simulink model "PID_simulink"  (R2025a)
settings: Solver=VariableStepAuto  StartTime=0.0  StopTime=10.0  RelTol=1e-3
undefined symbols (not defined in the file or in its folder): Kd1, Kd2, Ki1, Ki2, Kp1, Kp2
settings Model: Creator=j chandini gayathri  LastModifiedBy=j chandini gayathri

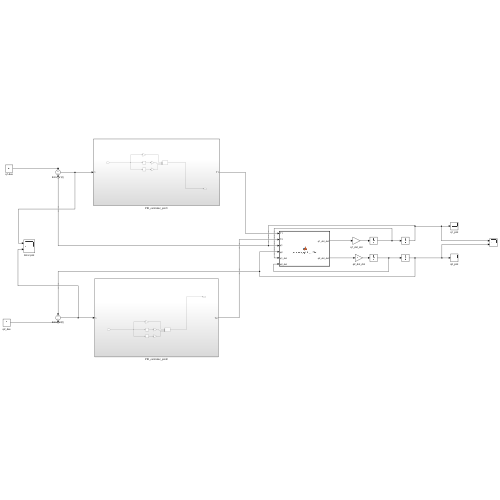
[thumbnail: Simulink's stored preview of the top-level diagram]
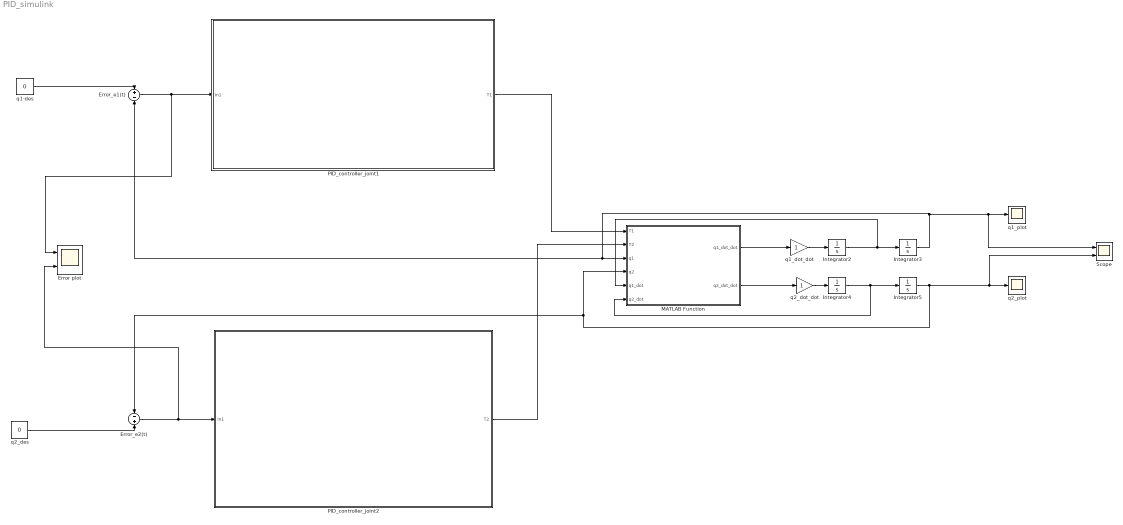
== system PID_simulink ==
  Error plot : Scope  NumInputPorts=2
      settings: Title=Ki_1= 5,Ki_2=5,Kp_1=200,Kp_2=200,Kd_1=400,Kd_2=400  ActiveDisplayYMinimum=-5.3633481280846287E+43  ActiveDisplayYMaximum=5.6403532247882645E+43  DataLoggingVariableName=ScopeData2
  Error_e1(t) : Sum  Inputs=+-
  Error_e2(t) : Sum  Inputs=-+
  Integrator{2..5} (4 alike) : Integrator
  MATLAB Function : MATLAB Function  TreatAsAtomicUnit=on
  PID_controller_joint1 : Subsystem
  PID_controller_joint2 : Subsystem
  Scope : Scope  NumInputPorts=2
      settings: ActiveDisplayYMinimum=-0.092497055065485209  ActiveDisplayYMaximum=0.011310468207808053  DataLoggingVariableName=ScopeData3
  q1-des : Constant  Value=0
  q1_dot_dot : Gain
  q1_plot : Scope
      settings: ActiveDisplayYMinimum=-0.092497055065485209  ActiveDisplayYMaximum=0.011310468207808053
  q2_des : Constant  Value=0
  q2_dot_dot : Gain
  q2_plot : Scope
      settings: ActiveDisplayYMinimum=-0.0028522802877235659  ActiveDisplayYMaximum=0.00045683308329411837
  wires:
  q1-des/1 -> Error_e1(t)/1
  Integrator2/1 -> MATLAB Function/5(q1_dot), Integrator3/1
  Integrator4/1 -> MATLAB Function/6(q2_dot), Integrator5/1
  Integrator3/1 -> Error_e1(t)/2, MATLAB Function/3(q1), Scope/1, q1_plot/1
  Integrator5/1 -> MATLAB Function/4(q2), Error_e2(t)/1, Scope/2, q2_plot/1
  q2_des/1 -> Error_e2(t)/2
  Error_e1(t)/1 -> Error plot/1, PID_controller_joint1/1(In1)
  Error_e2(t)/1 -> Error plot/2, PID_controller_joint2/1(In1)
  PID_controller_joint1/1(T1) -> MATLAB Function/1(T1)
  MATLAB Function/1(q1_dot_dot) -> q1_dot_dot/1
  MATLAB Function/2(q2_dot_dot) -> q2_dot_dot/1
  q1_dot_dot/1 -> Integrator2/1
  q2_dot_dot/1 -> Integrator4/1
  PID_controller_joint2/1(T2) -> MATLAB Function/2(T2)

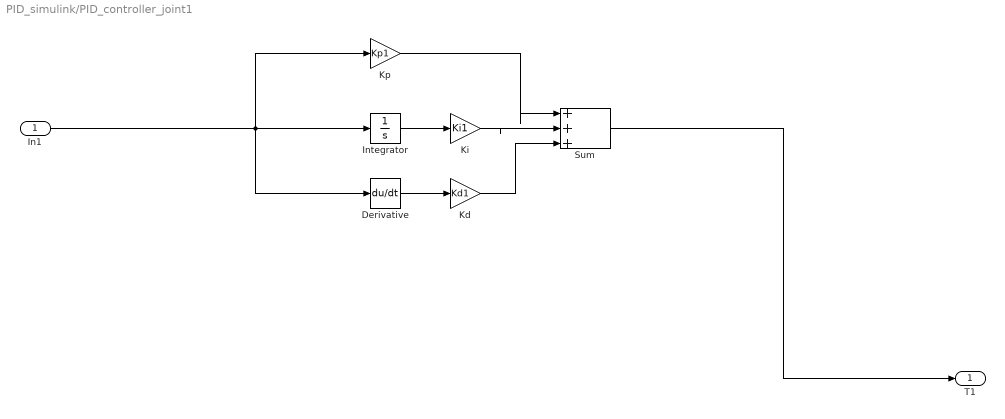
== system PID_simulink/PID_controller_joint1 ==
  In1 : Inport
  Derivative : Derivative
  Integrator : Integrator
  Kd : Gain  Gain=Kd1
  Ki : Gain  Gain=Ki1
  Kp : Gain  Gain=Kp1
  Sum : Sum  Inputs=|+++
  T1 : Outport
  wires:
  Kd/1 -> Sum/3
  Kp/1 -> Sum/1
  In1/1 -> Derivative/1, Kp/1, Integrator/1
  Derivative/1 -> Kd/1
  Sum/1 -> T1/1
  Integrator/1 -> Ki/1
  Ki/1 -> Sum/2

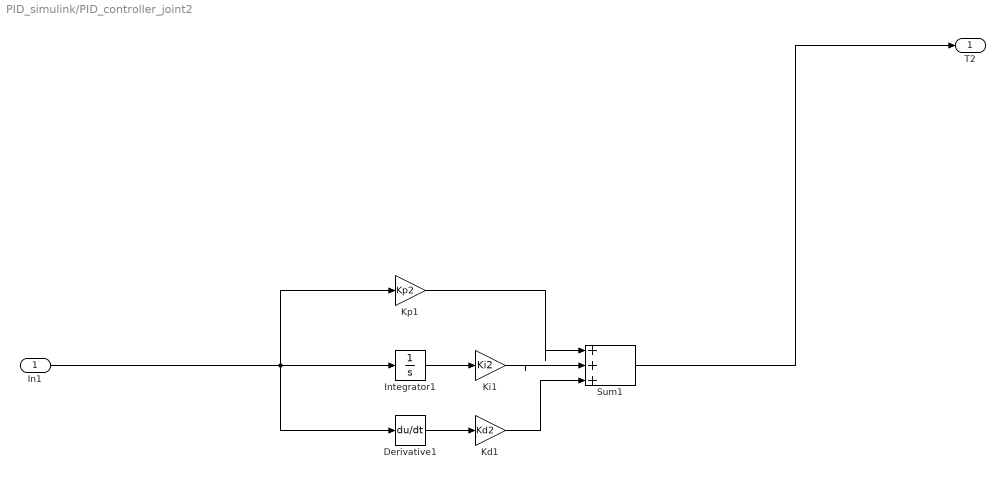
== system PID_simulink/PID_controller_joint2 ==
  In1 : Inport
  Derivative1 : Derivative
  Integrator1 : Integrator
  Kd1 : Gain  Gain=Kd2
  Ki1 : Gain  Gain=Ki2
  Kp1 : Gain  Gain=Kp2
  Sum1 : Sum  Inputs=|+++
  T2 : Outport
  wires:
  In1/1 -> Derivative1/1, Kp1/1, Integrator1/1
  Sum1/1 -> T2/1
  Kd1/1 -> Sum1/3
  Derivative1/1 -> Kd1/1
  Kp1/1 -> Sum1/1
  Ki1/1 -> Sum1/2
  Integrator1/1 -> Ki1/1

== matlab function PID_simulink/MATLAB Function ==
  data: T1 input; q1_dot_dot output; T2 input; q1 input; q2 input; q1_dot input; q2_dot input; q2_dot_dot output
function [q1_dot_dot, q2_dot_dot] = compute_q1dd_q2dd(T1, T2, q1, q2, q1_dot, q2_dot)
    m1 = 5; 
    m2 = 3;  
    l1 = 0.25; 
    l2 = 0.15; 
    g = 9.81; 
    M11 = (m1 + m2)*l1^2 + m2*l2*(l2 + 2*l1*cos(q2));
    M12=m2*l2*(l2 + l1*cos(q2));
    M21=m2*l2*(l2 + l1*cos(q2));
    M22=m2*l2^2;
    M=[M11 M12; M21 M22];
    C11 = -m2*l1*l2*sin(q2)*q2_dot;
    C12 = -m2*l1*l2*sin(q2)*(q1_dot + q2_dot);
    C21 = 0;
    C22 = m2*l1*l2*sin(q2)*q1_dot;
    C = [C11 C12; C21 C22];
    G1 = m1*l1*g*cos(q1) + m2*g*(l2*cos(q1 + q2) + l1*cos(q1));
    G2 = m2*g*l2*cos(q1 + q2);
    G = [G1; G2];
    tau = [T1; T2];
    q_dot = [q1_dot; q2_dot];
    q_dot_dot = (tau - (C*q_dot + G))./M;
    q1_dot_dot = q_dot_dot(1);
    q2_dot_dot = q_dot_dot(2);
end
